simulink model "TrayectoriaPurePursuit"  (R2023b)
settings: Solver=FixedStepDiscrete  StartTime=0.0  StopTime=200  FixedStep=0.01  MaxStep=0.01  RelTol=1e-3  EnableMultiTasking=on
model workspace (MAT data in the model file):
  d = 1
libraries: robotalgslib x1
settings Model: ExtModeTrigDuration=2  Creator=Usuario_UMA  LastModifiedBy=Daniel
settings OptimizationCC: EnhancedBackFolding=on  PassReuseOutputArgsAs=Individual arguments  ZeroExternalMemoryAtStartup=off  ZeroInternalMemoryAtStartup=off  MaxStackSize=64  OptimizeBlockOrder=speed  DifferentSizesBufferReuse=on  OptimizationCustomize=off  EfficientTunableParamExpr=on
settings DebuggingCC: ParameterTunabilityLossMsg=error
settings HardwareCC: ProdBitPerInt=16  ProdBitPerPointer=16  ProdBitPerSizeT=16  ProdBitPerPtrDiffT=16  ProdLargestAtomicFloat=None  ProdWordSize=8  ProdHWDeviceType=Atmel->AVR  UseEmbeddedCoderFeatures=off  UseSimulinkCoderFeatures=off
settings SFSimCC: MATLABDynamicMemAlloc=off
settings RTWCC: Description=Embedded Coder  SystemTargetFile=ert.tlc  HardwareBoard=Arduino Mega 2560  TemplateMakefile=ert_default_tmf  Toolchain=Arduino AVR  BuildConfiguration=Faster Runs
settings CodeAppCC: ForceParamTrailComments=on  IgnoreCustomStorageClasses=off  OperatorAnnotations=on  SimulinkDataObjDesc=on  SFDataObjDesc=on  InsertBlockDesc=on
settings ERTTargetCC: SupportContinuousTime=on  SupportNonInlinedSFcns=on  SupportVariableSizeSignals=on  ExtModeTransport=3  ExtModeStaticAlloc=on  ExtModeAutomaticAllocSize=off  ExtModeStaticAllocSize=2048  ExtModeMexFile=ext_xcp  ExtModeIntrfLevel=Level2 - Open

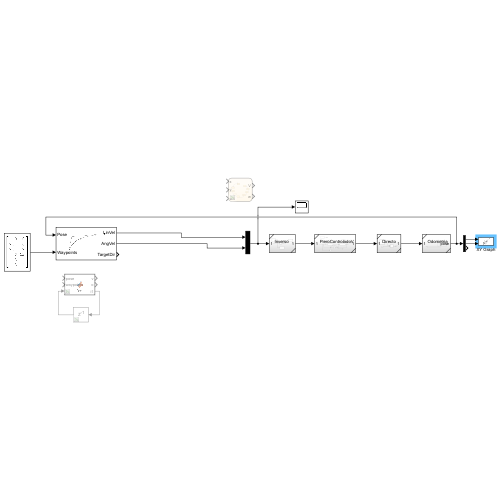
[thumbnail: Simulink's stored preview of the top-level diagram]
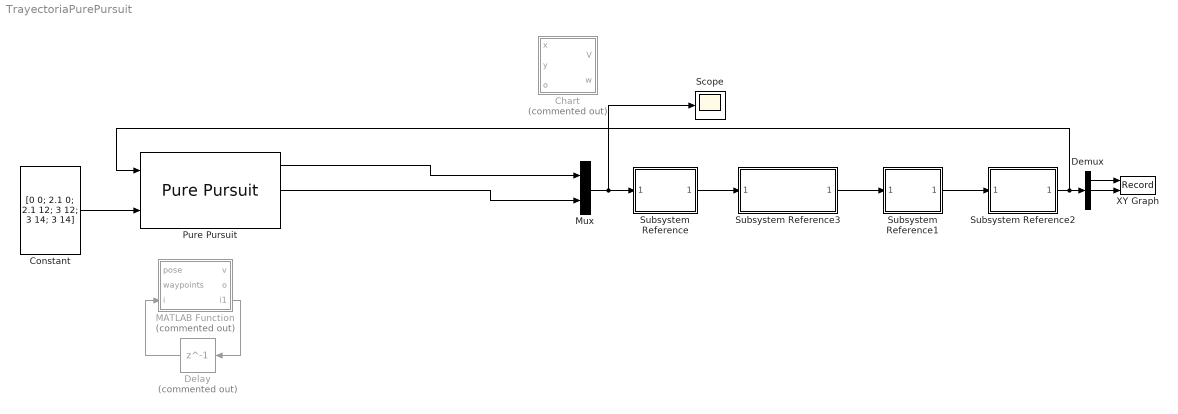
== system TrayectoriaPurePursuit ==
  Chart : Stateflow chart  Commented=on  TreatAsAtomicUnit=on
  Constant : Constant  Value=[0 0; 2.1 0; 2.1 12; 3 12; 3 14; 3 14]
  Delay : Delay  Commented=on  DelayLength=1
  Demux : Demux  Outputs=3
  MATLAB Function : MATLAB Function  Commented=on  TreatAsAtomicUnit=on
  Mux : Mux  Inputs=2
  Pure Pursuit : robotalgslib/Pure Pursuit  DesiredLinearVelocity=0.205  MaxAngularVelocity=0.75  LookaheadDistance=0.5  TargetDirPort=on  SimulateUsing=Code generation
      settings: LibrarySourceBlock=navlib/Control Algorithms/Pure Pursuit
  Scope : Scope
  Subsystem Reference : Subsystem  ReferencedSubsystem=Inverso
  Subsystem Reference1 : Subsystem  ReferencedSubsystem=Directo
  Subsystem Reference2 : Subsystem  ReferencedSubsystem=Odometria
  Subsystem Reference3 : Subsystem  ReferencedSubsystem=PieroControladoV
  XY Graph : Record  FileSettingsInternal="{\"entries\":[{\"content\":{\"excelSettings\":{\"content\":{},\"type\":\"Streamout.ExcelSettings\"}},\"type\":\"Streamout.FileSettingStorage\",\"uuid\":\"\"}],\"packageUris\":[\"http:\\/\\/schema.mathworks.com\\/mf0\\/streamout_blocks\\/R2020a\"],\"version\":\"1.0\"}"  Layout=[1 1]  SignalsInternal="{\"entries\":[{\"content\":{\"signals\":[{\"content\":{\"blockPath\":[],\"dimensions\":[1],\"domain\":\"\",\"lineColor\":\"#fe330a\",\"plots\":[ 1 ],\"port\":1,\"sid\":[\"\"],\"signalID\":1,\"signalName\":\"Demux:1\"},\"type\":\"RecordBlkView.Signal\",\"uuid\":\"\"},{\"content\":{\"blockPath\":[],\"dimensions\":[1],\"domain\":\"\",\"lineColor\":\"#22b573\",\"plots\":[ 1 ],\"port\":2,\"sid\":[\"\"],\"signalID\":2,\"signalName\":\"Demux:2\"},\"type\":\"RecordBlkView.Signal\",\"uuid\":\"\"}]},\"type\":\"RecordBlkView.InputSignals\",\"uuid\":\"\"}],\"packageUris\":[\"http:\\/\\/schema.mathworks.com\\/mf0\\/streamout_blocks\\/R2020a\"],\"version\":\"1.0\"}"  VisualizationBindings="{\"xyplotplugin\":{\"info\":[{\"series\":[{\"bindingParametersList\":[{\"parameter\":\"X-Axis\",\"signalID\":1,\"signalName\":\"Demux:1\"},{\"parameter\":\"Y-Axis\",\"signalID\":2,\"signalName\":\"Demux:2\"}],\"seriesID\":0}],\"subplotID\":1}]}}"  CompatibilityTag=XY
  wires:
  Subsystem Reference/1 -> Subsystem Reference3/1
  Subsystem Reference3/1 -> Subsystem Reference1/1
  Subsystem Reference1/1 -> Subsystem Reference2/1
  Subsystem Reference2/1 -> Pure Pursuit/1, Demux/1
  Demux/2 -> XY Graph/2
  Demux/1 -> XY Graph/1
  Mux/1 -> Scope/1, Subsystem Reference/1
  Pure Pursuit/2 -> Mux/2
  Pure Pursuit/1 -> Mux/1
  Constant/1 -> Pure Pursuit/2
  MATLAB Function/3(i1) -> Delay/1
  Delay/1 -> MATLAB Function/3(i)

== matlab function TrayectoriaPurePursuit/MATLAB Function ==
  data: pose input; v output; waypoints input; o output; i input; i1 output
function [v, o, i1] = fcn(pose, waypoints, i)
LA=0.30;
%if isempty (indice)
%   persistent indice=0;

v = 0.205;
i=i+1;
i1=0;
x=pose(1);
y=pose(2);
O=pose(3);

if(length(waypoints)>=i)
    distancia=sqrt((waypoints(i,1)-x)^2 +(waypoints(i,2)-x)^2);
    while (distancia<LA)&&(length(waypoints)<i)
        i=i+1;
        distancia=sqrt((waypoints(i,1)-x)^2 +(waypoints(i,2)-x)^2);
        v=0.1;
    end
    o=atan2(waypoints(i,2)-y,waypoints(i,1)-x);
else
    o=pose(3);
    v=0;
end
if(length(waypoints)>i)
    i1=i-1;
else
    i1=1;
end

== stateflow chart TrayectoriaPurePursuit/Chart ==
  state Inicio
    w=0;
    V=0;
  state Estado8
    w=pi/2;
    V=0;
  state Estado1
    w=0;
    V=0.205;
  state Estado7
    w=pi/2;
    V=0.205;
  state Estado2
    w=pi/2;
    V=0.1;
  state Estado6
    w=pi/2;
    V=0.1;
  state Estado3
    w=pi/2;
    V=0.205;
  state Estado5
    w=0;
    V=0.205;
  state Estado4
    w=0;
    V=0.1;
  (default) -> Inicio
  Inicio -> Estado1 : after (1, seconds)
  Estado7 -> Estado8 : [y<14]
  Estado1 -> Estado2 : [x>2.1]
  Estado6 -> Estado7 : [o>pi/2]
  Estado2 -> Estado3 : [o>pi/2]
  Estado5 -> Estado6 : [x>3]
  Estado3 -> Estado4 : [y>12]
  Estado4 -> Estado5 : [o>0]
  data: V output double size=1; w output double size=1; x input; y input; o input
